simulink model "simulink_38"  (R2023b)
settings: Solver=FixedStepAuto  StartTime=0.0  StopTime=10.0  FixedStep=1e-3  RelTol=1e-3  EnableMultiTasking=on
undefined symbols (not defined in the file): A0, A1, D0, D1, D10, D11, D12, D13, D2, D3, D4, D5, D6, D7, D8, D9, magnitude, PTA0, PTA1, PTA2, PTB2, PTB23, PTB3, PTB9, PTC16, PTC17, PTC2, PTC3, PTC4, PTD0, PTD1, PTD2, PTD3
libraries: frdmk64flib x23, etargetslib x16
settings Model: ExtModeTrigDuration=5  Creator=Harry Easton  LastModifiedBy=Harry Easton
settings SolverCC: AlgebraicLoopSolver=TrustRegion
settings OptimizationCC: EnhancedBackFolding=on  PassReuseOutputArgsAs=Individual arguments  ZeroExternalMemoryAtStartup=off  ZeroInternalMemoryAtStartup=off  MaxStackSize=64  OptimizeBlockOrder=speed  DifferentSizesBufferReuse=on  OptimizationCustomize=off  EfficientTunableParamExpr=on
settings DebuggingCC: ParameterTunabilityLossMsg=error  UnconnectedInputMsg=warning  UnconnectedOutputMsg=warning  UnconnectedLineMsg=warning
settings HardwareCC: ProdBitPerPointer=32  ProdBitPerSizeT=32  ProdBitPerPtrDiffT=32  ProdLargestAtomicInteger=Long  ProdLargestAtomicFloat=Double  ProdWordSize=32  ProdHWDeviceType=ARM Compatible->ARM Cortex
settings ModelReferenceCC: EnableRefExpFcnMdlSchedulingChecks=on
settings SFSimCC: MATLABDynamicMemAlloc=off
settings RTWCC: Description=Embedded Coder  SystemTargetFile=ert.tlc  HardwareBoard=NXP FRDM-K64F  TLCOptions="-aInlineSetEventsForThisBaseRateFcn=TLC_FALSE -aSuppressMultiTaskScheduler=TLC_FALSE  -aRateBasedStepFcn=0"  TemplateMakefile=ert_default_tmf  Toolchain=GNU Tools for ARM Embedded Processors
settings CodeAppCC: ForceParamTrailComments=on  IgnoreCustomStorageClasses=off  OperatorAnnotations=on  SimulinkDataObjDesc=on  SFDataObjDesc=on  InsertBlockDesc=on

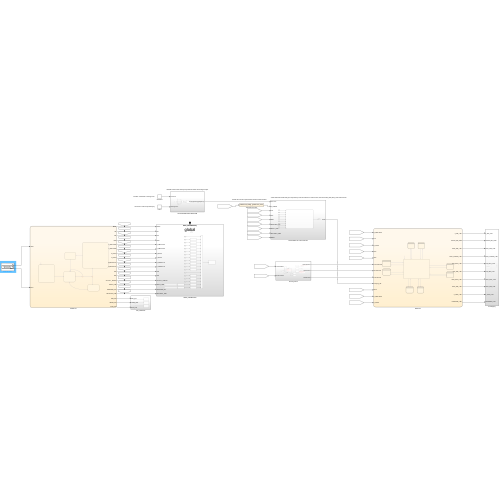
[thumbnail: Simulink's stored preview of the top-level diagram]
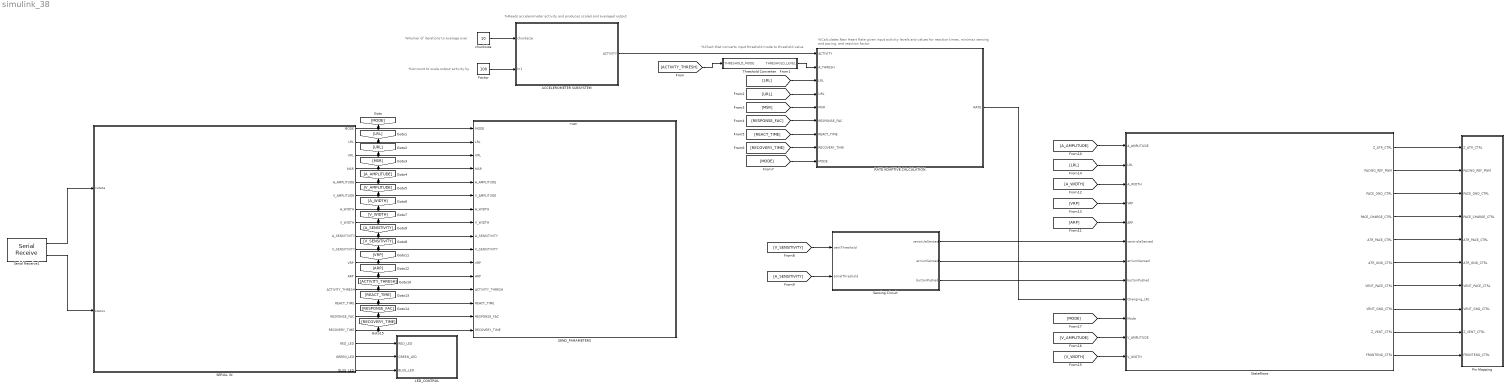
== system simulink_38 ==
  note: %Reads accelerometer activity and produces scaled and averaged output
  note: %Numer of iterations to average over
  note: %Chart that converts input threshold mode to threshold value
  note: %Calculates New Heart Rate given input activity levels and values for reaction times, min/max sensing and pacing, and reaction factor
  note: %Amount to scale output activity by
  ACCELEROMETER SUBSYSTEM : Subsystem
  Factor : Constant  Value=100
  LED_CONTROL : Subsystem
  Pin Mapping : Subsystem
  RATE ADAPTIVE CALCULATION : Subsystem
  SEND_PARAMETERS : Subsystem  TreatAsAtomicUnit=on
  SERIAL IN : Stateflow chart  TreatAsAtomicUnit=on
      settings: PortSchema="{\"entries\":[{\"content\":{\"sides\":[{\"content\":{\"connectorIds\":[\"In1\",\"In2\"]},\"type\":\"ConnectorPlacement.EquallySpacedRectSide\",\"uuid\":\"98fd8f1f-66ff-403c-bee2-89ad2f12b110\"},{\"content\":{\"connectorIds\":[\"Out8\",\"Out7\",\"Out14\",\"Out9\",\"Out2\",\"Out16\",\"Out4\",\"Out18\",\"Out3\",\"Out17\",\"Out15\",\"Out19\",\"Out1\",\"Out10\",\"Out13\",\"Out11\",\"Out12\",\"Out6\",\"Out5\"],\"side\":\"RIGHT\"},\"type\":\"ConnectorPlacement.EquallySpacedRectSide\",\"uuid\":\"01582ffe-c7e5-450d-a4ce-489c04458376\"},{\"content\":{\"side\":\"TOP\"},\"type\":\"ConnectorPlacement.EquallySpacedRectSide\",\"uuid\":\"dd9a8aa9-24f6-40f7-813c-a8e0a898beac\"}]},\"type\":\"ConnectorPlacement.EquallySpacedConnector\",\"uuid\":\"1011d1e7-27fc-459d-aa79-5cbb08dc9f7b\"}],\"packageUris\":[\"http://schema.mathworks.com/mf0/Connector/R2020b\"],\"version\":\"1.0\"}"
  Sensing Circuit : Subsystem
  Serial Receive1 : frdmk64flib/Serial Receive  SCIModule=0  Baudrate=uint32(9600)  Parity=None  StopBits=1  HardwareFlowControl=None  ByteOrder=LittleEndian  DataType=uint8  DataLength=40  BlockingMode=off  OutputStatus=on  SampleTime=-1
  Stateflows : Stateflow chart  TreatAsAtomicUnit=on
      settings: PortSchema="{\"entries\":[{\"content\":{\"sides\":[{\"content\":{\"connectorIds\":[\"In1\",\"In2\",\"In8\",\"In5\",\"In6\",\"In4\",\"In3\",\"In7\",\"In9\",\"In10\",\"In11\",\"In12\"]},\"type\":\"ConnectorPlacement.EquallySpacedRectSide\",\"uuid\":\"fd7a65b5-6a9e-486c-b395-8752d247d110\"},{\"content\":{\"connectorIds\":[\"Out1\",\"Out2\",\"Out3\",\"Out4\",\"Out5\",\"Out6\",\"Out7\",\"Out8\",\"Out9\",\"Out10\"],\"side\":\"RIGHT\"},\"type\":\"ConnectorPlacement.EquallySpacedRectSide\",\"uuid\":\"2771a934-b7e6-4717-9d0f-b17bdbdca872\"},{\"content\":{\"side\":\"TOP\"},\"type\":\"ConnectorPlacement.EquallySpacedRectSide\",\"uuid\":\"3a68066b-1574-4876-94b5-372b67bc25b8\"}]},\"type\":\"ConnectorPlacement.EquallySpacedConnector\",\"uuid\":\"cd95133d-7553-4814-ba78-1fbdc0c00507\"}],\"packageUris\":[\"http://schema.mathworks.com/mf0/Connector/R2020b\"],\"version\":\"1.0\"}"
  Threshold Converter : Stateflow chart  TreatAsAtomicUnit=on
  chunksize : Constant  Value=10
  wires:
  Stateflows/1(Z_ATR_CTRL) -> Pin Mapping/1(Z_ATR_CTRL)
  Stateflows/2(PACING_REF_PWM) -> Pin Mapping/2(PACING_REF_PWM)
  Stateflows/3(PACE_GND_CTRL) -> Pin Mapping/3(PACE_GND_CTRL)
  Stateflows/4(PACE_CHARGE_CTRL) -> Pin Mapping/4(PACE_CHARGE_CTRL)
  Stateflows/5(ATR_PACE_CTRL) -> Pin Mapping/5(ATR_PACE_CTRL)
  Stateflows/6(ATR_GND_CTRL) -> Pin Mapping/6(ATR_GND_CTRL)
  Stateflows/7(VENT_PACE_CTRL) -> Pin Mapping/7(VENT_PACE_CTRL)
  Stateflows/8(VENT_GND_CTRL) -> Pin Mapping/8(VENT_GND_CTRL)
  Stateflows/9(Z_VENT_CTRL) -> Pin Mapping/9(Z_VENT_CTRL)
  Stateflows/10(FRONTEND_CTRL) -> Pin Mapping/10(FRONTEND_CTRL)
  [LRL] -> Stateflows/2(LRL)
  [ARP] -> Stateflows/6(ARP)
  [MODE] -> Stateflows/10(Mode)
  [V_WIDTH] -> Stateflows/12(V_WIDTH)
  [A_SENSITIVITY] -> Sensing Circuit/2(atrialThreshold)
  [V_SENSITIVITY] -> Sensing Circuit/1(ventThreshold)
  Sensing Circuit/2(atriumSensed) -> Stateflows/3(atriumSensed)
  Sensing Circuit/1(ventricleSensed) -> Stateflows/4(ventricleSensed)
  Sensing Circuit/3(buttonPushed) -> Stateflows/7(buttonPushed)
  ACCELEROMETER SUBSYSTEM/1(ACTIVITY) -> RATE ADAPTIVE CALCULATION/1(ACTIVITY)
  chunksize/1 -> ACCELEROMETER SUBSYSTEM/1(chunksize)
  Factor/1 -> ACCELEROMETER SUBSYSTEM/2(In1)
  Threshold Converter/1(THRESHOLD_LEVEL) -> RATE ADAPTIVE CALCULATION/2(A_THRESH)
  [LRL] -> RATE ADAPTIVE CALCULATION/3(LRL)
  RATE ADAPTIVE CALCULATION/1(RATE) -> Stateflows/9(Changing_LRL)
  [V_AMPLITUDE] -> Stateflows/11(V_AMPLITUDE)
  SERIAL IN/13(RESPONSE_FAC) -> [RESPONSE_FAC], SEND_PARAMETERS/15(RESPONSE_FAC)
  Serial Receive1/1 -> SERIAL IN/1(rxdata)
  SERIAL IN/1(ACTIVITY_THRESH) -> [ACTIVITY_THRESH], SEND_PARAMETERS/13(ACTIVITY_THRESH)
  SERIAL IN/11(RECOVERY_TIME) -> [RECOVERY_TIME], SEND_PARAMETERS/16(RECOVERY_TIME)
  SERIAL IN/17(V_SENSITIVITY) -> [V_SENSITIVITY], SEND_PARAMETERS/10(V_SENSITIVITY)
  SERIAL IN/7(LRL) -> [LRL], SEND_PARAMETERS/2(LRL)
  SERIAL IN/19(ARP) -> [ARP], SEND_PARAMETERS/12(ARP)
  SERIAL IN/2(A_AMPLITUDE) -> [A_AMPLITUDE], SEND_PARAMETERS/5(A_AMPLITUDE)
  SERIAL IN/4(A_WIDTH) -> [A_WIDTH], SEND_PARAMETERS/7(A_WIDTH)
  Serial Receive1/2 -> SERIAL IN/2(status)
  SERIAL IN/12(RED_LED) -> LED_CONTROL/1(RED_LED)
  SERIAL IN/15(VRP) -> [VRP], SEND_PARAMETERS/11(VRP)
  SERIAL IN/8(MODE) -> [MODE], SEND_PARAMETERS/1(MODE)
  SERIAL IN/10(REACT_TIME) -> [REACT_TIME], SEND_PARAMETERS/14(REACT_TIME)
  SERIAL IN/14(URL) -> [URL], SEND_PARAMETERS/3(URL)
  SERIAL IN/5(BLUE_LED) -> LED_CONTROL/3(BLUE_LED)
  SERIAL IN/3(A_SENSITIVITY) -> [A_SENSITIVITY], SEND_PARAMETERS/9(A_SENSITIVITY)
  SERIAL IN/16(V_AMPLITUDE) -> [V_AMPLITUDE], SEND_PARAMETERS/6(V_AMPLITUDE)
  SERIAL IN/6(GREEN_LED) -> LED_CONTROL/2(GREEN_LED)
  SERIAL IN/18(V_WIDTH) -> [V_WIDTH], SEND_PARAMETERS/8(V_WIDTH)
  SERIAL IN/9(MSR) -> [MSR], SEND_PARAMETERS/4(MSR)
  [ACTIVITY_THRESH] -> Threshold Converter/1(THRESHOLD_MODE)
  [URL] -> RATE ADAPTIVE CALCULATION/4(URL)
  [MSR] -> RATE ADAPTIVE CALCULATION/5(MSR)
  [RESPONSE_FAC] -> RATE ADAPTIVE CALCULATION/6(RESPONSE_FAC)
  [REACT_TIME] -> RATE ADAPTIVE CALCULATION/7(REACT_TIME)
  [RECOVERY_TIME] -> RATE ADAPTIVE CALCULATION/8(RECOVERY_TIME)
  [MODE] -> RATE ADAPTIVE CALCULATION/9(MODE)
  [VRP] -> Stateflows/5(VRP)
  [A_AMPLITUDE] -> Stateflows/1(A_AMPLITUDE)
  [A_WIDTH] -> Stateflows/8(A_WIDTH)

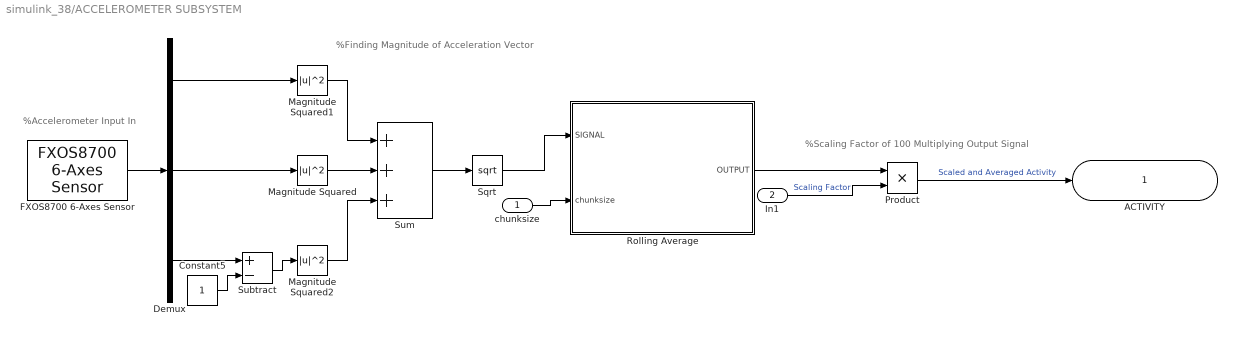
== system simulink_38/ACCELEROMETER SUBSYSTEM ==
  note: %Scaling Factor of 100 Multiplying Output Signal
  note: %Finding Magnitude of Acceleration Vector
  note: %Accelerometer Input In
  chunksize : Inport
  In1 : Inport  Port=2
  Constant5 : Constant
  Demux : Demux  Outputs=3
  FXOS8700 6-Axes Sensor : frdmk64flib/FXOS8700 6-Axes Sensor  Activesensor=Accelerometer only  ODR=800Hz  HybridODR=400Hz  Accelfullrange=-4g to +4g  SampleTime=0.01
  Magnitude Squared : Math  Operator=magnitude^2
  Magnitude Squared1 : Math  Operator=magnitude^2
  Magnitude Squared2 : Math  Operator=magnitude^2
  Product : Product
  Rolling Average : Stateflow chart  TreatAsAtomicUnit=on
  Sqrt : Sqrt  IntermediateResultsDataTypeStr=double
  Subtract : Sum  Inputs=+-
  Sum : Sum  Inputs=+++
  ACTIVITY : Outport
  wires:
  Rolling Average/1(OUTPUT) -> Product/1
  Sum/1 -> Sqrt/1
  Demux/1 -> Magnitude Squared1/1
  Sqrt/1 -> Rolling Average/1(SIGNAL)
  FXOS8700 6-Axes Sensor/1 -> Demux/1
  Demux/2 -> Magnitude Squared/1
  Subtract/1 -> Magnitude Squared2/1
  Constant5/1 -> Subtract/2
  Magnitude Squared/1 -> Sum/2
  Magnitude Squared2/1 -> Sum/3
  Magnitude Squared1/1 -> Sum/1
  Demux/3 -> Subtract/1
  In1/1 -> Product/2  "Scaling Factor"
  Product/1 -> ACTIVITY/1  "Scaled and Averaged Activity"
  chunksize/1 -> Rolling Average/2(chunksize)

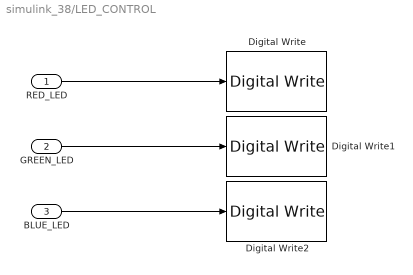
== system simulink_38/LED_CONTROL ==
  RED_LED : Inport
  GREEN_LED : Inport  Port=2
  BLUE_LED : Inport  Port=3
  Digital Write : frdmk64flib/Digital Write  Whichpin=RED_LED
  Digital Write1 : frdmk64flib/Digital Write  Whichpin=GREEN_LED
  Digital Write2 : frdmk64flib/Digital Write  Whichpin=BLUE_LED
  wires:
  RED_LED/1 -> Digital Write/1
  GREEN_LED/1 -> Digital Write1/1
  BLUE_LED/1 -> Digital Write2/1

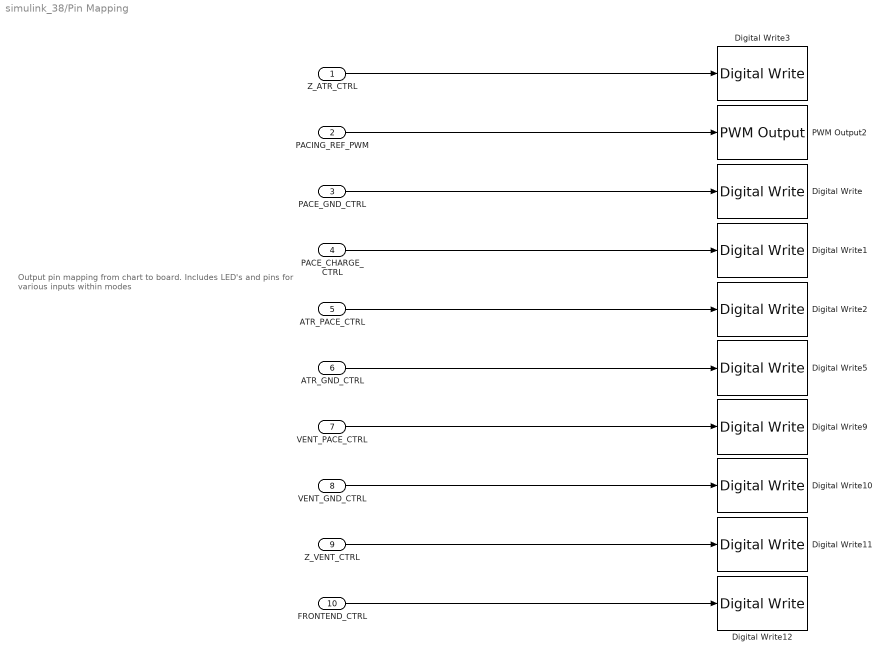
== system simulink_38/Pin Mapping ==
  note: Output pin mapping from chart to board.
      | Includes LED's and pins for various
      | inputs within modes
  Z_ATR_CTRL : Inport
  PACING_REF_PWM : Inport  Port=2
  PACE_GND_CTRL : Inport  Port=3
  PACE_CHARGE_CTRL : Inport  Port=4
  ATR_PACE_CTRL : Inport  Port=5
  ATR_GND_CTRL : Inport  Port=6
  VENT_PACE_CTRL : Inport  Port=7
  VENT_GND_CTRL : Inport  Port=8
  Z_VENT_CTRL : Inport  Port=9
  FRONTEND_CTRL : Inport  Port=10
  Digital Write : frdmk64flib/Digital Write  Whichpin=PTD0 (D10)
  Digital Write1 : frdmk64flib/Digital Write  Whichpin=PTB9 (D2)
  Digital Write10 : frdmk64flib/Digital Write  Whichpin=PTD3 (D12)
  Digital Write11 : frdmk64flib/Digital Write  Whichpin=PTC3 (D7)
  Digital Write12 : frdmk64flib/Digital Write  Whichpin=PTD1 (D13)
  Digital Write2 : frdmk64flib/Digital Write  Whichpin=PTA0 (D8)
  Digital Write3 : frdmk64flib/Digital Write  Whichpin=PTB23 (D4)
  Digital Write5 : frdmk64flib/Digital Write  Whichpin=PTD2 (D11)
  Digital Write9 : frdmk64flib/Digital Write  Whichpin=PTC4 (D9)
  PWM Output2 : frdmk64flib/PWM Output  Whichpin=PTA2 (D5)  InitialFrequency=2000  InitialDutyCycle=0
  wires:
  Z_ATR_CTRL/1 -> Digital Write3/1
  PACING_REF_PWM/1 -> PWM Output2/1
  PACE_CHARGE_CTRL/1 -> Digital Write1/1
  ATR_GND_CTRL/1 -> Digital Write5/1
  ATR_PACE_CTRL/1 -> Digital Write2/1
  PACE_GND_CTRL/1 -> Digital Write/1
  Z_VENT_CTRL/1 -> Digital Write11/1
  VENT_PACE_CTRL/1 -> Digital Write9/1
  VENT_GND_CTRL/1 -> Digital Write10/1
  FRONTEND_CTRL/1 -> Digital Write12/1

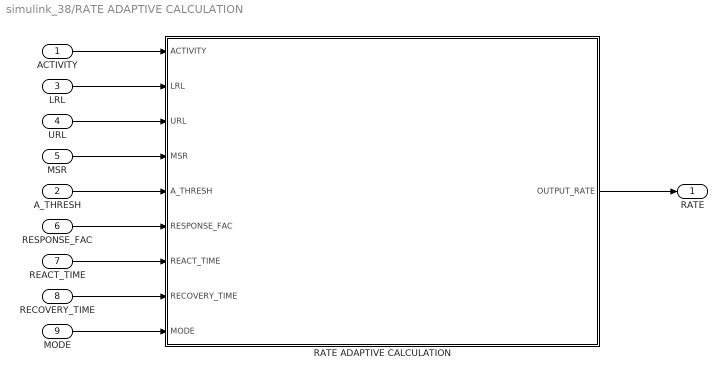
== system simulink_38/RATE ADAPTIVE CALCULATION ==
  ACTIVITY : Inport
  A_THRESH : Inport  Port=2
  LRL : Inport  Port=3
  URL : Inport  Port=4
  MSR : Inport  Port=5
  RESPONSE_FAC : Inport  Port=6
  REACT_TIME : Inport  Port=7
  RECOVERY_TIME : Inport  Port=8
  MODE : Inport  Port=9
  RATE ADAPTIVE CALCULATION : Stateflow chart  TreatAsAtomicUnit=on
  RATE : Outport  OutDataTypeStr=uint16
  wires:
  LRL/1 -> RATE ADAPTIVE CALCULATION/2(LRL)
  REACT_TIME/1 -> RATE ADAPTIVE CALCULATION/7(REACT_TIME)
  MSR/1 -> RATE ADAPTIVE CALCULATION/4(MSR)
  RECOVERY_TIME/1 -> RATE ADAPTIVE CALCULATION/8(RECOVERY_TIME)
  A_THRESH/1 -> RATE ADAPTIVE CALCULATION/5(A_THRESH)
  RESPONSE_FAC/1 -> RATE ADAPTIVE CALCULATION/6(RESPONSE_FAC)
  RATE ADAPTIVE CALCULATION/1(OUTPUT_RATE) -> RATE/1
  ACTIVITY/1 -> RATE ADAPTIVE CALCULATION/1(ACTIVITY)
  URL/1 -> RATE ADAPTIVE CALCULATION/3(URL)
  MODE/1 -> RATE ADAPTIVE CALCULATION/9(MODE)

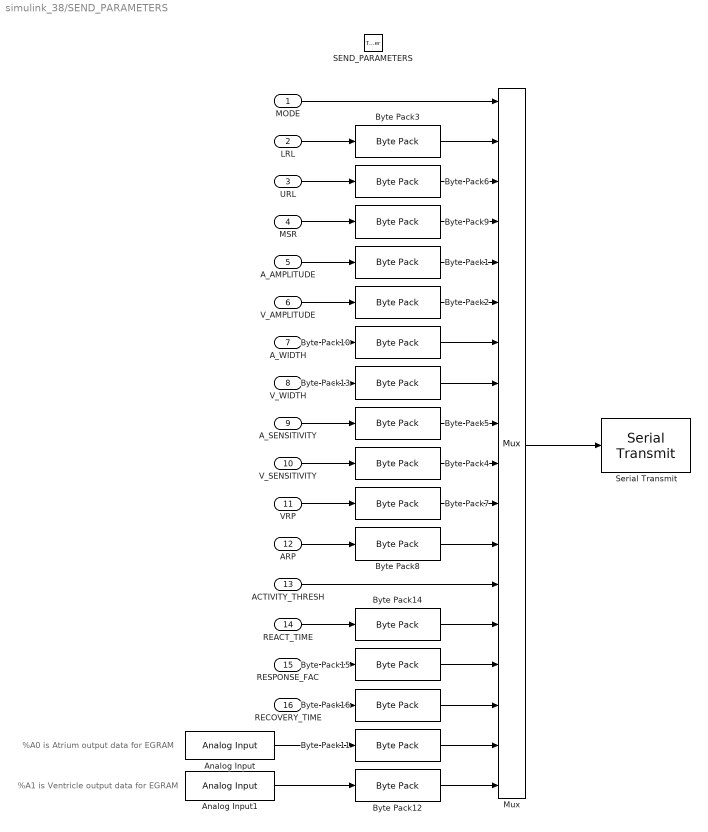
== system simulink_38/SEND_PARAMETERS ==
  note: %A1 is Ventricle output data for EGRAM
  note: %A0 is Atrium output data for EGRAM
  MODE : Inport  OutDataTypeStr=uint8
  LRL : Inport  Port=2  OutDataTypeStr=uint16
  URL : Inport  Port=3  OutDataTypeStr=uint16
  MSR : Inport  Port=4  OutDataTypeStr=uint16
  A_AMPLITUDE : Inport  Port=5  OutDataTypeStr=single
  V_AMPLITUDE : Inport  Port=6  OutDataTypeStr=single
  A_WIDTH : Inport  Port=7  OutDataTypeStr=uint16
  V_WIDTH : Inport  Port=8  OutDataTypeStr=uint16
  A_SENSITIVITY : Inport  Port=9  OutDataTypeStr=single
  V_SENSITIVITY : Inport  Port=10  OutDataTypeStr=single
  VRP : Inport  Port=11  OutDataTypeStr=uint16
  ARP : Inport  Port=12  OutDataTypeStr=uint16
  ACTIVITY_THRESH : Inport  Port=13  OutDataTypeStr=uint8
  REACT_TIME : Inport  Port=14  OutDataTypeStr=uint16
  RESPONSE_FAC : Inport  Port=15  OutDataTypeStr=uint16
  RECOVERY_TIME : Inport  Port=16  OutDataTypeStr=uint16
  SEND_PARAMETERS : TriggerPort  TriggerType=function-call  IsSimulinkFunction=on  FunctionName=SEND_PARAMETERS  VariantControl=(inherit)
  Analog Input : frdmk64flib/Analog Input  Whichpin=PTB2 (A0)  SampleTime=-1
  Analog Input1 : frdmk64flib/Analog Input  Whichpin=PTB3 (A1)  SampleTime=-1
  Byte Pack{1..2,4..5} (4 alike) : etargetslib/Byte Pack  datatypes={'single'}  byteAlign=1
  Byte Pack{3,6..10,13..16} (10 alike) : etargetslib/Byte Pack  datatypes={'uint16'}  byteAlign=1
  Byte Pack11 : etargetslib/Byte Pack  datatypes={'double'}  byteAlign=1
  Byte Pack12 : etargetslib/Byte Pack  datatypes={'double'}  byteAlign=1
  Mux : Mux  Inputs=18
  Serial Transmit : frdmk64flib/Serial Transmit  SCIModule=0  Baudrate=uint32(9600)  Parity=None  StopBits=1  HardwareFlowControl=None  ByteOrder=LittleEndian  BlockingMode=on  OutputStatus=off
  wires:
  A_AMPLITUDE/1 -> Byte Pack1/1
  V_AMPLITUDE/1 -> Byte Pack2/1
  A_SENSITIVITY/1 -> Byte Pack5/1
  V_SENSITIVITY/1 -> Byte Pack4/1
  VRP/1 -> Byte Pack7/1
  ARP/1 -> Byte Pack8/1
  Mux/1 -> Serial Transmit/1
  MODE/1 -> Mux/1
  Byte Pack1/1 -> Mux/5
  Byte Pack2/1 -> Mux/6
  Byte Pack5/1 -> Mux/9
  Byte Pack4/1 -> Mux/10
  Byte Pack7/1 -> Mux/11
  Byte Pack8/1 -> Mux/12
  ACTIVITY_THRESH/1 -> Mux/13
  Analog Input1/1 -> Byte Pack12/1
  Analog Input/1 -> Byte Pack11/1
  Byte Pack11/1 -> Mux/17
  Byte Pack12/1 -> Mux/18
  LRL/1 -> Byte Pack3/1
  Byte Pack3/1 -> Mux/2
  Byte Pack6/1 -> Mux/3
  Byte Pack9/1 -> Mux/4
  URL/1 -> Byte Pack6/1
  MSR/1 -> Byte Pack9/1
  A_WIDTH/1 -> Byte Pack10/1
  Byte Pack10/1 -> Mux/7
  Byte Pack13/1 -> Mux/8
  V_WIDTH/1 -> Byte Pack13/1
  REACT_TIME/1 -> Byte Pack14/1
  Byte Pack14/1 -> Mux/14
  RESPONSE_FAC/1 -> Byte Pack15/1
  Byte Pack15/1 -> Mux/15
  RECOVERY_TIME/1 -> Byte Pack16/1
  Byte Pack16/1 -> Mux/16

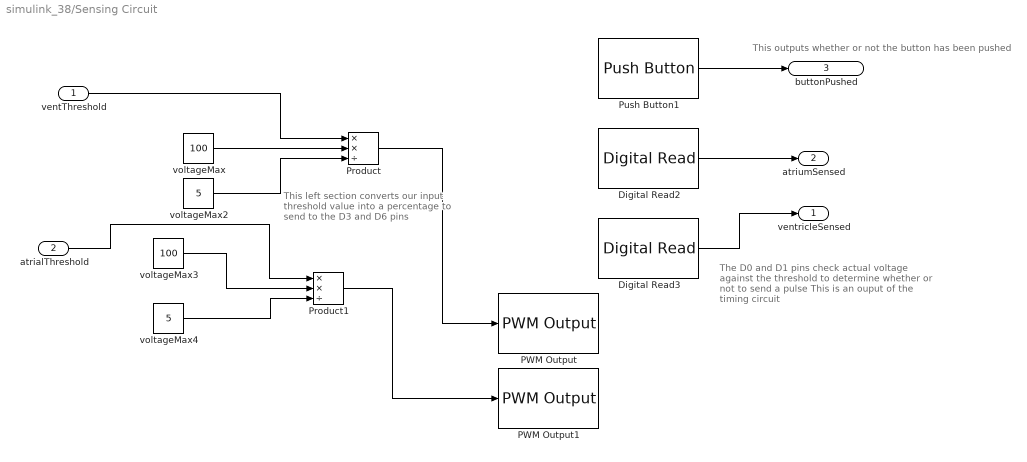
== system simulink_38/Sensing Circuit ==
  note: This outputs whether or not the button has been pushed
  note: The D0 and D1 pins check actual voltage
      | against the threshold to determine whether
      | or not to send a pulse
      | This is an ouput of the timing circuit
  note: This left section converts our input threshold value
      | into a percentage to send to the D3 and D6 pins
  ventThreshold : Inport
  atrialThreshold : Inport  Port=2
  Digital Read2 : frdmk64flib/Digital Read  Whichpin=PTC16 (D0)  SampleTime=-1
  Digital Read3 : frdmk64flib/Digital Read  Whichpin=PTC17 (D1)  SampleTime=-1
  PWM Output : frdmk64flib/PWM Output  Whichpin=PTA1 (D3)  InitialFrequency=2000  InitialDutyCycle=0
  PWM Output1 : frdmk64flib/PWM Output  Whichpin=PTC2 (D6)  InitialFrequency=2000  InitialDutyCycle=0
  Product : Product  Inputs=**/
  Product1 : Product  Inputs=**/
  Push Button1 : frdmk64flib/Push Button  Whichswitch=SW2  SampleTime1=-1
  voltageMax : Constant  Value=100
  voltageMax2 : Constant  Value=5
  voltageMax3 : Constant  Value=100
  voltageMax4 : Constant  Value=5
  ventricleSensed : Outport
  atriumSensed : Outport  Port=2
  buttonPushed : Outport  Port=3
  wires:
  atrialThreshold/1 -> Product1/1
  voltageMax3/1 -> Product1/2
  ventThreshold/1 -> Product/1
  voltageMax/1 -> Product/2
  Product1/1 -> PWM Output1/1
  Product/1 -> PWM Output/1
  voltageMax2/1 -> Product/3
  Digital Read2/1 -> atriumSensed/1
  Digital Read3/1 -> ventricleSensed/1
  Push Button1/1 -> buttonPushed/1
  voltageMax4/1 -> Product1/3

== stateflow chart simulink_38/SERIAL IN ==
  settings: executeAtInitialization=1
  state SET_PARAMETERS
    entry:
    %rxdata(1) is ready for transmit
    %rxdata(2) is send or receive
    MODE = rxdata(3);
    LRL = typecast(rxdata(4:5), 'uint16');
    URL = typecast(rxdata(6:7), 'uint16');
    MSR = typecast(rxdata(8:9), 'uint16');
    A_AMPLITUDE = typecast(rxdata(10:13), 'single');
    V_AMPLITUDE = typecast(rxdata(14:17), 'single');
    A_WIDTH = typecast(rxdata(18:19), 'uint16');
    V_WIDTH = typecast(rxdata(20:21), 'uint16');
    A_SENSITIVITY = typecast(rxdata(22:25), 'single');
    V_SENSITIVITY = typecast(rxdata(26:29), 'single');
    VRP = typecast(rxdata(30:31), 'uint16');
    ARP = typecast(rxdata(32:33), 'uint16');
    ACTIVITY_THRESH = rxdata(34);
    REACT_TIME = typecast(rxdata(35:36), 'uint16');
    RESPONSE_FAC = typecast(rxdata(37:38), 'uint16');
    RECOVERY_TIME = typecast(rxdata(39:40), 'uint16');
    RED_LED = uint8(1); %Flash RED LED to signal params updated
  state SEND_PARAMETERS
    entry:
    SEND_PARAMETERS();
    GREEN_LED = uint8(1);
    %Flash GREEN LED to
    %signal params confirmed
  state INITIAL
    entry:
    MODE = uint8(1); %int from 1-8
    LRL = uint16(60); %bpm
    URL = uint16(120); %bpm
    MSR = uint16(120); %bpm
    A_AMPLITUDE = single(5); %V
    V_AMPLITUDE = single(5); %V
    A_WIDTH = uint16(1); %ms
    V_WIDTH = uint16(1); %ms
    A_SENSITIVITY = single(3); %mV
    V_SENSITIVITY = single(3); %mV
    VRP = uint16(320); %ms
    ARP = uint16(250); %ms
    ACTIVITY_THRESH = uint8(3); %int 0-6
    REACT_TIME = uint16(30); %sec
    RESPONSE_FAC = uint16(8); %int
    RECOVERY_TIME = uint16(5); %min
  state STANDBY
    %Waiting for COM
    RED_LED = 0;
    GREEN_LED = 0;
    BLUE_LED = 0;
  state SEND_EGRAM
    entry:
    SEND_PARAMETERS()
    BLUE_LED = uint8(1);
    %Flash BLUE LED to signal
    %data sent for EGRAM
  SET_PARAMETERS -> SEND_PARAMETERS
  SEND_PARAMETERS -> STANDBY
  (default) -> INITIAL
  (junction 22) -> SET_PARAMETERS [order 1] : [rxdata(2) == hex2dec('01')]
      | %Receive Data
  (junction 13) -> STANDBY [order 2]
  INITIAL -> STANDBY
  STANDBY -> (junction 13) : [status == 0]
  (junction 13) -> (junction 22) [order 1] : [rxdata(1) == hex2dec('00')]
      | % Beginning of Transmission
  (junction 22) -> SEND_EGRAM [order 2] : [rxdata(2) == hex2dec('02')]
      | %Send EGram
  SEND_EGRAM -> STANDBY
  data: rxdata input uint8; status input uint8; ACTIVITY_THRESH output uint8; A_AMPLITUDE output single; A_SENSITIVITY output single; A_WIDTH output uint16; BLUE_LED output uint8; GREEN_LED output uint8; LRL output uint16; MODE output uint8; MSR output uint16; REACT_TIME output uint16; RECOVERY_TIME output uint16; RED_LED output uint8; RESPONSE_FAC output uint16; URL output uint16; VRP output uint16; V_AMPLITUDE output single; V_SENSITIVITY output single; V_WIDTH output uint16; ARP output uint16

== stateflow chart simulink_38/ACCELEROMETER SUBSYSTEM/Rolling Average ==
  state OUTPUT_STATE
    %Get average, set output to new average
    entry:
    %get average of total, based off number of iterations
    total = total/COUNTER;
    OUTPUT = total;
    %Output is maintained till next accumulation completes
  state ACCUMULATE
    entry:
    %Constantly accumulates input value of signals
    %Adds current value of signal every iteration
    total = total + SIGNAL;
    COUNTER = COUNTER + 1;
    %Increase count of singals accumulated
  note: %wait until specified cycles to average completes
  (default) -> ACCUMULATE : {COUNTER=0, total=0}
  OUTPUT_STATE -> ACCUMULATE : {COUNTER = 0, total = 0}
  ACCUMULATE -> ACCUMULATE [order 2] : [COUNTER < chunksize]
  ACCUMULATE -> OUTPUT_STATE [order 1] : [COUNTER >= chunksize]
  data: COUNTER local; total local; SIGNAL input; OUTPUT output; chunksize input

== stateflow chart simulink_38/Stateflows ==
  state VOO
    state Charging
      % parameters laid out by documentation for Charging
      entry:
      PACING_REF_PWM = (V_AMPLITUDE/5)*100;
      PACE_GND_CTRL = 1;
      ATR_GND_CTRL = 0;
      VENT_GND_CTRL = 1;
      PACE_CHARGE_CTRL = 1;
      Z_VENT_CTRL = 0;
      ATR_GND_CTRL
      VENT_PACE_CTRL = 0;
      Pulse_Period = (60000/LRL);
    state Pacing
      % parameters laid out by documentation for Pacing
      entry:
      PACING_REF_PWM = (V_AMPLITUDE/5)*100;
      VENT_PACE_CTRL = 1;
      VENT_GND_CTRL = 0;
      PACE_CHARGE_CTRL = 0;
      PACE_GND_CTRL = 1;
      Z_VENT_CTRL = 0;
    note: Ventricular pacing, no sensing
    (default) -> VOO.Charging
    VOO.Charging -> VOO.Pacing : [after(Pulse_Period-V_WIDTH,msec)]
    VOO.Pacing -> VOO.Charging : [after(V_WIDTH,msec)]
  state AOO
    note: Atrial pacing, no sensing
    state Charging1
      % parameters laid out by documentation for Charging
      entry:
      PACING_REF_PWM = (A_AMPLITUDE/5)*100;
      PACE_CHARGE_CTRL = 1;
      ATR_PACE_CTRL = 0;
      VENT_PACE_CTRL = 0;
      PACE_GND_CTRL = 1;
      ATR_GND_CTRL = 1;
      VENT_GND_CTRL = 0;
      Z_ATR_CTRL = 0;
      Pulse_Period = (60000/LRL);
    state Pacing1
      % parameters laid out by documentation for Pacing
      entry:
      PACING_REF_PWM = (A_AMPLITUDE/5)*100;
      PACE_CHARGE_CTRL = 0;
      PACE_GND_CTRL = 1;
      ATR_PACE_CTRL = 1;
      ATR_GND_CTRL = 0;
      Z_ATR_CTRL = 0;
    (default) -> AOO.Charging1
    AOO.Charging1 -> AOO.Pacing1 : [after(Pulse_Period-A_WIDTH,msec)]
    AOO.Pacing1 -> AOO.Charging1 : [after(A_WIDTH,msec)]
  state Start
  state AAIR
    state Charging3
      % parameters laid out by documentation for Charging
      entry:
      PACING_REF_PWM = (A_AMPLITUDE/5)*100;
      PACE_CHARGE_CTRL=1;
      ATR_PACE_CTRL= 0;
      VENT_PACE_CTRL = 0;
      ATR_GND_CTRL= 1;
      VENT_GND_CTRL = 0;
      PACE_GND_CTRL=1;
      Z_ATR_CTRL=0;
      FRONTEND_CTRL = 1;
      Changing_Rate = (60000/Changing_LRL);
    state Pacing3
      % parameters laid out by documentation for Pacing
      entry:
      PACING_REF_PWM = (A_AMPLITUDE/5)*100;
      PACE_CHARGE_CTRL=0;
      ATR_PACE_CTRL= 1;
      ATR_GND_CTRL= 0;
      PACE_GND_CTRL=1;
      Z_ATR_CTRL=0;
    state Refractor_and_Sensing
    note: Atrial pacing, atrial sensing, sensed intrinsic signal inhibits atrial pacing, Rate Adaptive Mode
    (default) -> AAIR.Charging3
    AAIR.Refractor_and_Sensing -> AAIR.Charging3 [order 1] : [atriumSensed == 1 | buttonPushed == true]
    AAIR.Refractor_and_Sensing -> AAIR.Pacing3 [order 2] : after(Changing_Rate-ARP-A_WIDTH,msec)[atriumSensed == 0 & buttonPushed == false]
    AAIR.Charging3 -> AAIR.Refractor_and_Sensing : after(ARP, msec)
    AAIR.Pacing3 -> AAIR.Charging3 : after(A_WIDTH,msec)
  state AAI
    state Pacing3
      % parameters laid out by documentation for Pacing
      entry:
      PACING_REF_PWM = (A_AMPLITUDE/5)*100;
      PACE_CHARGE_CTRL=0;
      ATR_PACE_CTRL= 1;
      ATR_GND_CTRL= 0;
      PACE_GND_CTRL=1;
      Z_ATR_CTRL=0;
    state Charging3
      % parameters laid out by documentation for Charging
      entry:
      PACING_REF_PWM = (A_AMPLITUDE/5)*100;
      PACE_CHARGE_CTRL=1;
      ATR_PACE_CTRL= 0;
      VENT_PACE_CTRL = 0;
      ATR_GND_CTRL= 1;
      VENT_GND_CTRL = 0;
      PACE_GND_CTRL=1;
      Z_ATR_CTRL=0;
      FRONTEND_CTRL = 1;
      Pulse_Period = (60000/LRL);
    state Refractor_and_Sensing
    note: Atrial pacing, atrial sensing, sensed intrinsic signal inhibits atrial pacing
    (default) -> AAI.Charging3
    AAI.Refractor_and_Sensing -> AAI.Charging3 [order 1] : [atriumSensed == 1 | buttonPushed == true]
    AAI.Refractor_and_Sensing -> AAI.Pacing3 [order 2] : after(Pulse_Period-ARP-A_WIDTH,msec)[atriumSensed == 0 & buttonPushed == false]
    AAI.Charging3 -> AAI.Refractor_and_Sensing : after(ARP, msec)
    AAI.Pacing3 -> AAI.Charging3 : after(A_WIDTH,msec)
  state VVIR
    note: Ventricular pacing, ventricular sensing, sensed intrinsic signal inhibits ventricular pacing, Rate Adaptive Mode
    state Pacing2
      % parameters laid out by documentation for Pacing
      entry:
      PACE_CHARGE_CTRL = 0;
      PACE_GND_CTRL = 1;
      Z_VENT_CTRL = 0;
      VENT_GND_CTRL = 0;
      VENT_PACE_CTRL = 1;
    state Charging2
      % parameters laid out by documentation for Charging
      entry:
      FRONTEND_CTRL = 1;
      PACING_REF_PWM = (V_AMPLITUDE/5)*100;
      ATR_PACE_CTRL = 0;
      VENT_PACE_CTRL = 0;
      PACE_CHARGE_CTRL = 1;
      PACE_GND_CTRL = 1;
      Z_VENT_CTRL = 0;
      ATR_GND_CTRL = 0;
      VENT_GND_CTRL = 1;
      Changing_Rate = (60000/Changing_LRL);
    state Refractor_and_Sensing
    (default) -> VVIR.Charging2
    VVIR.Pacing2 -> VVIR.Charging2 : [after(V_WIDTH,msec)]
    VVIR.Refractor_and_Sensing -> VVIR.Pacing2 [order 2] : after(Changing_Rate-VRP-V_WIDTH,msec)[ventricleSensed == 0 & buttonPushed == false]
    VVIR.Charging2 -> VVIR.Refractor_and_Sensing : after(VRP,msec)
    VVIR.Refractor_and_Sensing -> VVIR.Charging2 [order 1] : [ventricleSensed == 1 | buttonPushed == true]
  state VVI
    note: Ventricular pacing, ventricular sensing, sensed intrinsic signal inhibits ventricular pacing
    state Pacing2
      % parameters laid out by documentation for Pacing
      entry:
      PACE_CHARGE_CTRL = 0;
      PACE_GND_CTRL = 1;
      Z_VENT_CTRL = 0;
      VENT_GND_CTRL = 0;
      VENT_PACE_CTRL = 1;
    state Charging2
      % parameters laid out by documentation for Charging
      entry:
      FRONTEND_CTRL = 1;
      PACING_REF_PWM = (V_AMPLITUDE/5)*100;
      ATR_PACE_CTRL = 0;
      VENT_PACE_CTRL = 0;
      PACE_CHARGE_CTRL = 1;
      PACE_GND_CTRL = 1;
      Z_VENT_CTRL = 0;
      ATR_GND_CTRL = 0;
      VENT_GND_CTRL = 1;
      Pulse_Period = (60000/LRL);
    state Refractor_and_Sensing
    (default) -> VVI.Charging2
    VVI.Pacing2 -> VVI.Charging2 : [after(V_WIDTH,msec)]
    VVI.Refractor_and_Sensing -> VVI.Pacing2 [order 2] : after(Pulse_Period-VRP-V_WIDTH,msec)[ventricleSensed == 0 & buttonPushed == false]
    VVI.Charging2 -> VVI.Refractor_and_Sensing : after(VRP,msec)
    VVI.Refractor_and_Sensing -> VVI.Charging2 [order 1] : [ventricleSensed == 1 | buttonPushed == true]
  state VOOR
    state Charging
      % parameters laid out by documentation for Charging
      entry:
      PACING_REF_PWM = (V_AMPLITUDE/5)*100;
      PACE_CHARGE_CTRL = 1;
      ATR_PACE_CTRL = 0;
      VENT_PACE_CTRL = 0;
      PACE_GND_CTRL = 1;
      Z_VENT_CTRL = 0;
      ATR_GND_CTRL = 0;
      VENT_GND_CTRL = 1;
      Changing_Rate = (60000/Changing_LRL);
    state Pacing
      % parameters laid out by documentation for Pacing
      entry:
      PACING_REF_PWM = (V_AMPLITUDE/5)*100;
      PACE_CHARGE_CTRL = 0;
      PACE_GND_CTRL = 1;
      Z_VENT_CTRL = 0;
      VENT_GND_CTRL = 0;
      VENT_PACE_CTRL = 1;
    note: Ventricular pacing, no sensing; Rate Adaptive Mode
    (default) -> VOOR.Charging
    VOOR.Charging -> VOOR.Pacing : [after(Changing_Rate-V_WIDTH,msec)]
    VOOR.Pacing -> VOOR.Charging : [after(V_WIDTH,msec)]
  state AOOR
    note: Atrial pacing, no sensing; Rate Adaptive Mode
    state Charging1
      % parameters laid out by documentation for Charging
      entry:
      PACING_REF_PWM = (A_AMPLITUDE/5)*100;
      PACE_CHARGE_CTRL = 1;
      ATR_PACE_CTRL = 0;
      VENT_PACE_CTRL = 0;
      PACE_GND_CTRL = 1;
      ATR_GND_CTRL = 1;
      VENT_GND_CTRL = 0;
      Z_ATR_CTRL = 0;
      Changing_Rate = (60000/Changing_LRL);
    state Pacing1
      % parameters laid out by documentation for Pacing
      entry:
      PACING_REF_PWM = (A_AMPLITUDE/5)*100;
      PACE_CHARGE_CTRL = 0;
      PACE_GND_CTRL = 1;
      ATR_PACE_CTRL = 1;
      ATR_GND_CTRL = 0;
      Z_ATR_CTRL = 0;
    (default) -> AOOR.Charging1
    AOOR.Charging1 -> AOOR.Pacing1 : [after(Changing_Rate-A_WIDTH,msec)]
    AOOR.Pacing1 -> AOOR.Charging1 : [after(A_WIDTH,msec)]
  Start -> AOO [order 4] : [Mode == 3]
  AOO -> Start : [Mode ~= 3]
  VOO -> Start : [Mode ~= 1]
  Start -> VOO [order 1] : [Mode == 1]
  (default) -> Start
  AAIR -> Start : [Mode ~= 8]
  Start -> AAIR [order 8] : [Mode == 8]
  Start -> AAI [order 5] : [Mode == 4]
  AAI -> Start : [Mode ~= 4]
  VVIR -> Start : [Mode ~= 6]
  Start -> VVIR [order 3] : [Mode == 6]
  VVI -> Start : [Mode ~= 2]
  Start -> VVI [order 2] : [Mode == 2]
  Start -> AOOR [order 7] : [Mode == 7]
  AOOR -> Start : [Mode ~= 7]
  VOOR -> Start : [Mode ~= 5]
  Start -> VOOR [order 6] : [Mode == 5]
  data: A_AMPLITUDE input single; LRL input uint16; atriumSensed input boolean; ventricleSensed input boolean; VRP input uint16; ARP input uint16; buttonPushed input boolean; A_WIDTH input uint16; Z_ATR_CTRL output; PACING_REF_PWM output; PACE_GND_CTRL output; PACE_CHARGE_CTRL output; ATR_PACE_CTRL output; ATR_GND_CTRL output; VENT_PACE_CTRL output; VENT_GND_CTRL output; Z_VENT_CTRL output; FRONTEND_CTRL output; Changing_LRL input uint16; Mode input uint8; V_AMPLITUDE input single; V_WIDTH input uint16; Pulse_Period local uint16; Changing_Rate local uint16

== stateflow chart simulink_38/RATE ADAPTIVE CALCULATION/RATE ADAPTIVE CALCULATION ==
  note: %100ms delay to avoid limitations. Rate is increased by 100 step increments accordingly.
  state RATE_CALCULATION
    %Calculate steps to increment and decrement per cycle
    %Convert to ms
    entry:
    STEP_REACTION = (double(MSR)-double(LRL))/(double(REACT_TIME)*1000);
    STEP_RECOVERY = (double(MSR)-double(LRL))/(double(RECOVERY_TIME)*60000);
    %Increases or decreases rate by min step
    %Multiplying by 100 due to 100msec delay
    if RATE < TARGET
    RATE = RATE + 100*STEP_REACTION;
    end
    if RATE > TARGET
    RATE = RATE - 100*STEP_RECOVERY;
    end
  state END
    entry:
    if MODE == 1 | MODE == 2 | MODE == 3 | MODE == 4
    RATE = double(LRL);
    end
    OUTPUT_RATE = uint16(RATE);
  state START
  state SLOPE_CALCULATION
    %SLOPE CALCULATION STATE
    %Calculates slope in slope variable
    %Calculates desired target depending on input activity
    entry:
    slope = (double(RESPONSE_FAC)/(10*double(MSR)) * (double(MSR) - A_THRESH));
    %Calculates the target rate based off the slope
    %Treating Threshold and LRL as origin
    TARGET = double(slope*(ACTIVITY - A_THRESH) + double(LRL));
    %Check Min and Max
    if (TARGET > double(MSR))
    TARGET = double(MSR);
    end
    if (TARGET > double(URL))
    TARGET = double(URL);
    end
    if (TARGET < double(LRL))
    TARGET = double(LRL)
    end
  END -> START : after(100, msec)
  START -> SLOPE_CALCULATION
  (default) -> START : {RATE = double(LRL), OUTPUT_RATE = LRL}
  SLOPE_CALCULATION -> RATE_CALCULATION
  RATE_CALCULATION -> END
  data: ACTIVITY input double; LRL input uint16; URL input uint16; MSR input uint16; slope local double; A_THRESH input double; RESPONSE_FAC input uint16; REACT_TIME input uint16; RECOVERY_TIME input uint16; MODE input uint8; RATE local double; OUTPUT_RATE output uint16; TARGET local; STEP_REACTION local; STEP_RECOVERY local

== stateflow chart simulink_38/Threshold Converter ==
  note: %chart converts enumerated instance to actual value
  state V_Low_Threshold
    entry:
    THRESHOLD_LEVEL = 20;
  state Low_Threshold
    entry:
    THRESHOLD_LEVEL = 40;
  state Med_Low_Threshold
    entry:
    THRESHOLD_LEVEL = 60;
  state Med_Threshold
    entry:
    THRESHOLD_LEVEL = 80;
  state EXIT1
  state Med_High_Threshold
    entry:
    THRESHOLD_LEVEL = 100;
  state High_Threshold
    entry:
    THRESHOLD_LEVEL = 120;
  state V_High_Threshold
    entry:
    THRESHOLD_LEVEL = 150;
  state EXIT
  EXIT1 -> (junction 1)
  (default) -> (junction 1) : {THRESHOLD_LEVEL = double(9)}
  V_Low_Threshold -> EXIT1
  (junction 1) -> V_Low_Threshold [order 1] : [THRESHOLD_MODE == 0]
  EXIT -> (junction 1)
  (junction 1) -> (junction 15) [order 2]
  (junction 15) -> Low_Threshold [order 1] : [THRESHOLD_MODE == 1]
  Low_Threshold -> EXIT1
  (junction 15) -> (junction 16) [order 2]
  (junction 16) -> Med_Low_Threshold [order 1] : [THRESHOLD_MODE == 2]
  Med_Low_Threshold -> EXIT1
  (junction 16) -> (junction 19) [order 2]
  (junction 19) -> Med_Threshold [order 1] : [THRESHOLD_MODE == 3]
  Med_Threshold -> EXIT1
  (junction 19) -> (junction 22) [order 2]
  V_High_Threshold -> EXIT1
  Med_High_Threshold -> EXIT1
  High_Threshold -> EXIT1
  (junction 22) -> Med_High_Threshold [order 1] : [THRESHOLD_MODE == 4]
  (junction 22) -> (junction 25) [order 2]
  (junction 25) -> High_Threshold [order 1] : [THRESHOLD_MODE == 5]
  (junction 25) -> (junction 28) [order 2]
  (junction 28) -> V_High_Threshold [order 1] : [THRESHOLD_MODE == 6]
  (junction 28) -> EXIT [order 2]
  data: THRESHOLD_MODE input; THRESHOLD_LEVEL output
